simulink model "lab2_sinusoidal_input"  (R2019b)
settings: Solver=FixedStepAuto  StartTime=0.0  StopTime=70.0  RelTol=1e-3  EnableMultiTasking=on
libraries: arduinolib x4
settings Model: SILPILModeSetting=veronly  ExtModeTrigDuration=2  Creator=MSI  LastModifiedBy=Dilek
settings OptimizationCC: EnhancedBackFolding=on  PassReuseOutputArgsAs=Individual arguments  ZeroExternalMemoryAtStartup=off  ZeroInternalMemoryAtStartup=off  MaxStackSize=64  OptimizeBlockOrder=speed  DifferentSizesBufferReuse=on  OptimizationCustomize=off  EfficientTunableParamExpr=on
settings DebuggingCC: ParameterTunabilityLossMsg=error
settings HardwareCC: ProdBitPerInt=16  ProdBitPerPointer=16  ProdBitPerSizeT=16  ProdBitPerPtrDiffT=16  ProdLargestAtomicFloat=None  ProdWordSize=8  ProdHWDeviceType=Atmel->AVR  UseEmbeddedCoderFeatures=off
settings SFSimCC: MATLABDynamicMemAlloc=off
settings RTWCC: SystemTargetFile=ert.tlc  HardwareBoard=Arduino Uno  TLCOptions=-aInlineSetEventsForThisBaseRateFcn=TLC_FALSE -aSuppressMultiTaskScheduler=TLC_FALSE -aRateBasedStepFcn=1  TemplateMakefile=ert_default_tmf  GenerateReport=on  Toolchain=Arduino AVR  BuildConfiguration=Faster Runs  IncludeHyperlinkInReport=on  LaunchReport=on  GenerateTraceInfo=on  GenerateTraceReport=on  GenerateTraceReportSl=on  GenerateTraceReportSf=on  GenerateTraceReportEml=on
settings CodeAppCC: ForceParamTrailComments=on  IgnoreCustomStorageClasses=off  OperatorAnnotations=on  SimulinkDataObjDesc=on  SFDataObjDesc=on  InsertBlockDesc=on
settings ERTTargetCC: SupportContinuousTime=on  SupportNonInlinedSFcns=on  SupportVariableSizeSignals=on  ExtModeStaticAllocSize=250

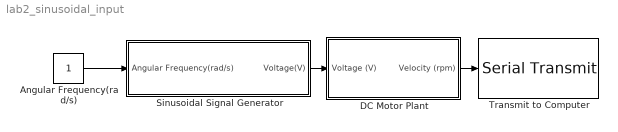
== system lab2_sinusoidal_input ==
  Angular Frequency(rad/s) : Constant
  DC Motor Plant : Subsystem
  Sinusoidal Signal Generator : Subsystem
  Transmit to Computer : arduinolib/Serial Transmit  portNumber=0  sendmode=write  sendformat=Decimal  floatprecision=2  blockPlatform=arduino
      settings: SourceProductName=Simulink Support Package for Arduino Hardware
  wires:
  DC Motor Plant/1(Velocity (rpm)) -> Transmit to Computer/1
  Angular Frequency(rad/s)/1 -> Sinusoidal Signal Generator/1(Angular Frequency(rad/s))
  Sinusoidal Signal Generator/1(Voltage(V)) -> DC Motor Plant/1(Voltage (V))

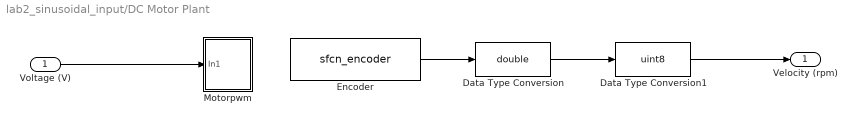
== system lab2_sinusoidal_input/DC Motor Plant ==
  Voltage (V) : Inport
  Data Type Conversion : DataTypeConversion  OutDataTypeStr=double
  Data Type Conversion1 : DataTypeConversion  OutDataTypeStr=uint8
  Encoder : S-Function  InitFcn=try, set_param(gcb,'FunctionName','sfcn_encoder'), end  FunctionName=sfcn_encoder  Parameters=uint8(0),uint8(2),uint8(3)  SFunctionModules=sfcn_encoder_wrapper  SFunctionDeploymentMode=off  EnableBusSupport=off  mask(S-Function Builder){}
      mask init:
      | val = [[.9  0.75 0.75 1 1 .9 .9 1]',[1 1 0.75 0.75 .9 .9 1 .9]'];try , sys = get_param(gcb,'SfunBuilderFcnName');if isempty(sys), sys = get_param(gcb,'FunctionName'); end,catch, sys = get_param(gcb,'FunctionName'); end
      settings: CopyFcn=set_param(gcbh,'LinkStatus','none')  PreSaveFcn=try, set_param(gcb,'FunctionName','sfcn_encoder'), end  OpenFcn=sfunctionwizard(gcbh)
      mask Display: plot(val(:,1),val(:,2)),disp(sys), port_label('output',1,'pos')
  Motorpwm : Subsystem
  Velocity (rpm) : Outport
  wires:
  Encoder/1 -> Data Type Conversion/1
  Voltage (V)/1 -> Motorpwm/1(In1)
  Data Type Conversion/1 -> Data Type Conversion1/1
  Data Type Conversion1/1 -> Velocity (rpm)/1

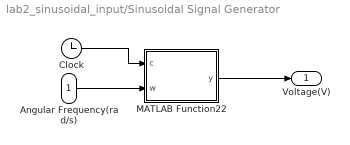
== system lab2_sinusoidal_input/Sinusoidal Signal Generator ==
  Angular Frequency(rad/s) : Inport
  Clock : Clock
  MATLAB Function22 : MATLAB Function  TreatAsAtomicUnit=on
  Voltage(V) : Outport
  wires:
  Clock/1 -> MATLAB Function22/1(c)
  MATLAB Function22/1(y) -> Voltage(V)/1
  Angular Frequency(rad/s)/1 -> MATLAB Function22/2(w)

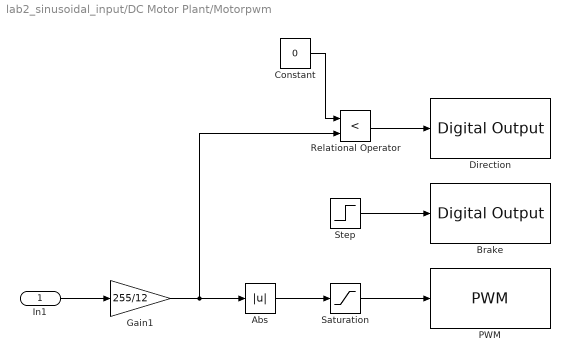
== system lab2_sinusoidal_input/DC Motor Plant/Motorpwm ==
  In1 : Inport
  Abs : Abs
  Brake : arduinolib/Digital Output  pinNumber=8  blockPlatform=arduino
  Constant : Constant  Value=0
  "Direction " : arduinolib/Digital Output  pinNumber=13  blockPlatform=arduino
  Gain1 : Gain  Gain=255/12
  PWM : arduinolib/PWM  pinNumber=11  EnableInputFrequency=off  InitialFrequency=2000  InitialDutyCycle=0  NotificationType=None  blockPlatform=arduino
  Relational Operator : RelationalOperator  Operator=<  OutDataTypeStr=boolean  RndMeth=Simplest
  Saturation : Saturate  UpperLimit=255  LowerLimit=0
  Step : Step  Time=0  After=0  SampleTime=0
  wires:
  Relational Operator/1 -> "Direction "/1
  Step/1 -> Brake/1
  Saturation/1 -> PWM/1
  In1/1 -> Gain1/1
  Abs/1 -> Saturation/1
  Constant/1 -> Relational Operator/1
  Gain1/1 -> Relational Operator/2, Abs/1

== matlab function lab2_sinusoidal_input/Sinusoidal Signal Generator/MATLAB Function22 ==
  data: y output; c input; w input
function y = fcn2(c,w)
%#codegen
if w<1
    scale=70;
elseif w<10
    scale=25;
else
    scale=10;
end   
 
if c<scale
    y = 10*sin(w*c);
else
    y=0;
end
